simulink subsystem "edge2x1_simple_asSubsystem"  (R2021a)
settings: Solver=VariableStepAuto  StartTime=0.0  StopTime=10.0  RelTol=1e-3
libraries: EdgesLibrary x2
settings Model: Creator=phill  LastModifiedBy=phill

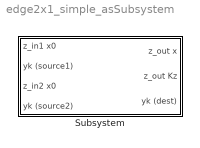
== system edge2x1_simple_asSubsystem ==
  Subsystem : Subsystem  mask{Rk1=0, Rk2=0.5}
      mask prompts: Rk1 "Rk (input 1)"; Rk2 "Rk (input 2)"
      settings: PortSchema="{\"entries\":[{\"content\":{\"sides\":[{\"content\":{\"connectorIds\":[\"In1\",\"Out2\",\"In2\",\"Out3\"]},\"type\":\"ConnectorPlacement.EquallySpacedRectSide\",\"uuid\":\"eb102e1f-8f68-4819-b192-9ed8ea7965cd\"},{\"content\":{\"connectorIds\":[\"In3\",\"In4\",\"Out1\"],\"side\":\"RIGHT\"},\"type\":\"ConnectorPlacement.EquallySpacedRectSide\",\"uuid\":\"0a8d41cc-2128-49e0-9ce9-20439c8bfca2\"},{\"content\":{\"connectorIds\":[],\"side\":\"TOP\"},\"type\":\"ConnectorPlacement.EquallySpacedRectSide\",\"uuid\":\"ce1e229b-7216-4f3c-b1ef-7720ca51f1c4\"}]},\"type\":\"ConnectorPlacement.EquallySpacedConnector\",\"uuid\":\"c8e8c67c-b38f-484f-95e7-011277152545\"}],\"packageUris\":[\"http://schema.mathworks.com/mf0/Connector/R2020b\"],\"version\":\"1.0\"}"
      mask Display:
      | image('$imagefile'); % Use "Edit Image" on toolstrip to change.
      | disp('Simple Edge 2x1\n\n\n');
      | Rk1 = get_param(gcb,'Rk1');
      | Rk2 = get_param(gcb, 'Rk2');
      | disp(['Rk1 = ', Rk1, ' | Rk2 =  ', Rk2])

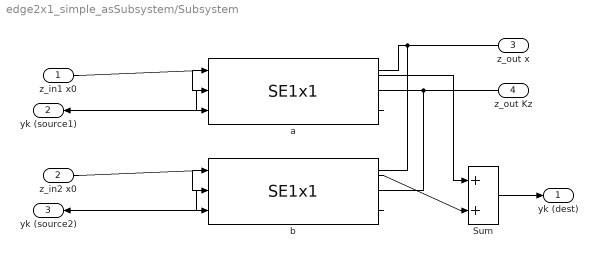
== system edge2x1_simple_asSubsystem/Subsystem ==
  z_in1 x0 : Inport
  z_in2 x0 : Inport  Port=2
  z_out x : Inport  Port=3
  z_out Kz : Inport  Port=4
  Sum : Sum
  a : EdgesLibrary/SE1x1  Rk=Rk1
  b : EdgesLibrary/SE1x1  Rk=Rk2
  yk (dest) : Outport
  yk (source1) : Outport  Port=2
  yk (source2) : Outport  Port=3
  wires:
  z_out Kz/1 -> b/3, a/3
  Sum/1 -> yk (dest)/1
  z_out x/1 -> b/2, a/2
  b/1 -> Sum/2
  z_in1 x0/1 -> a/1
  a/1 -> Sum/1
  z_in2 x0/1 -> b/1
  b/2 -> yk (source2)/1
  a/2 -> yk (source1)/1
